simulink model "Amplitude_Shift_Keying"  (R2024a)
settings: Solver=VariableStepAuto  StartTime=0.0  StopTime=10.0  RelTol=1e-3
libraries: commdigbbndapm x1
settings Model: Creator=online  LastModifiedBy=online
settings RTWCC: GPUComputeCapability=3.5

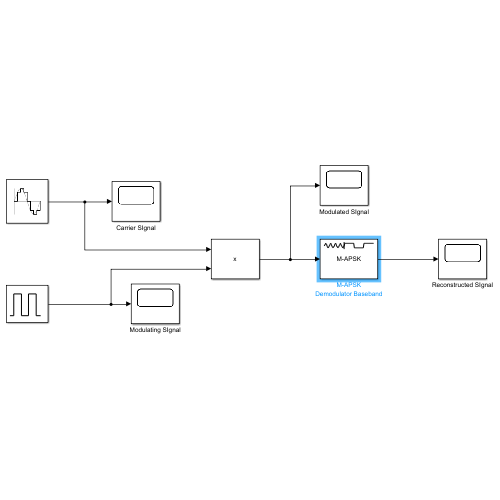
[thumbnail: Simulink's stored preview of the top-level diagram]
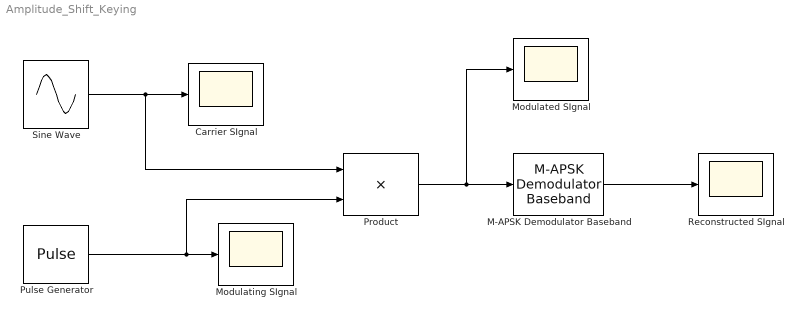
== system Amplitude_Shift_Keying ==
  Carrier SIgnal : Scope
  M-APSK Demodulator Baseband : commdigbbndapm/M-APSK Demodulator Baseband  ConstPointsCirclewise=[ 4, 12 ]  Radii=[ 0.5, 1 ]  PhaseOffset=[ pi/4, pi/12 ]  SymbolMapping=Auto  CustomSymbolMapping=[ 0, 4, 12, 8, 1, 3, 2, 6, 7, 5, 13, 15, 14, 10, 11, 9 ]  OutputType=Integer  DecisionType=Hard decision  VarianceSource=Property  NoiseVariance=1  OutputDataType=double  SimulateUsing=Interpreted execution
  Modulated SIgnal : Scope
  Modulating SIgnal : Scope
  Product : Product
  Pulse Generator : DiscretePulseGenerator  PulseType=Time based  Amplitude=0.5  PulseWidth=50
  Reconstructed SIgnal : Scope
  Sine Wave : Sin  Frequency=50  SampleTime=0.00001
  wires:
  Sine Wave/1 -> Carrier SIgnal/1, Product/1
  Pulse Generator/1 -> Modulating SIgnal/1, Product/2
  M-APSK Demodulator Baseband/1 -> Reconstructed SIgnal/1
  Product/1 -> Modulated SIgnal/1, M-APSK Demodulator Baseband/1
